simulink model "NucleoRespirator"  (R2018b)
settings: Solver=FixedStepDiscrete  StartTime=0.0  StopTime=10.0  FixedStep=MdlTS  RelTol=1e-3  SampleTimeConstraint=Specified  EnableMultiTasking=on
undefined symbols (not defined in the file): eSupervisorStates, NLCDDisplayColumns, ReleaseVersionMajor, ReleaseVersionMinor, ReleaseVersionRevision, tControlPeriod, tDisplayUpdatePeriode
libraries: RespiratorCtrlLib x37, simulink x4, LIB_Control x1
settings Model: DataDictionary=RespiratorControlData.sldd  ExtModeTrigDuration=10  Creator=BRAUL  LastModifiedBy=BRAUL
settings OptimizationCC: EnhancedBackFolding=on  PassReuseOutputArgsAs=Individual arguments  MaxStackSize=64  OptimizeBlockOrder=speed  DifferentSizesBufferReuse=on  OptimizationCustomize=off
settings DebuggingCC: UnderspecifiedInitializationDetection=Classic  MergeDetectMultiDrivingBlocksExec=none  ParameterTunabilityLossMsg=error
settings HardwareCC: ProdBitPerPointer=32  ProdBitPerSizeT=32  ProdBitPerPtrDiffT=32  ProdLargestAtomicInteger=Long  ProdLargestAtomicFloat=Double  ProdWordSize=32  ProdHWDeviceType=ARM Compatible->ARM Cortex
settings ModelReferenceCC: PropagateSignalLabelsOutOfModel=off
settings SFSimCC: MATLABDynamicMemAlloc=off
settings RTWCC: SystemTargetFile=ert.tlc  HardwareBoard=STM32 Nucleo F411RE  PackageGeneratedCodeAndArtifacts=on  TemplateMakefile=ert_default_tmf  GenerateReport=on  Toolchain=GNU Tools for ARM Embedded Processors  BuildConfiguration=Faster Runs  IncludeHyperlinkInReport=on  LaunchReport=on  GenerateTraceInfo=on  GenerateTraceReport=on  GenerateTraceReportSl=on  GenerateTraceReportSf=on  GenerateTraceReportEml=on  GenerateCodeReplacementReport=on
settings CodeAppCC: ForceParamTrailComments=on  IgnoreCustomStorageClasses=off  OperatorAnnotations=on  SimulinkDataObjDesc=on  SFDataObjDesc=on  InsertBlockDesc=on
settings ERTTargetCC: TargetLangStandard=C99 (ISO)  GenerateASAP2=on

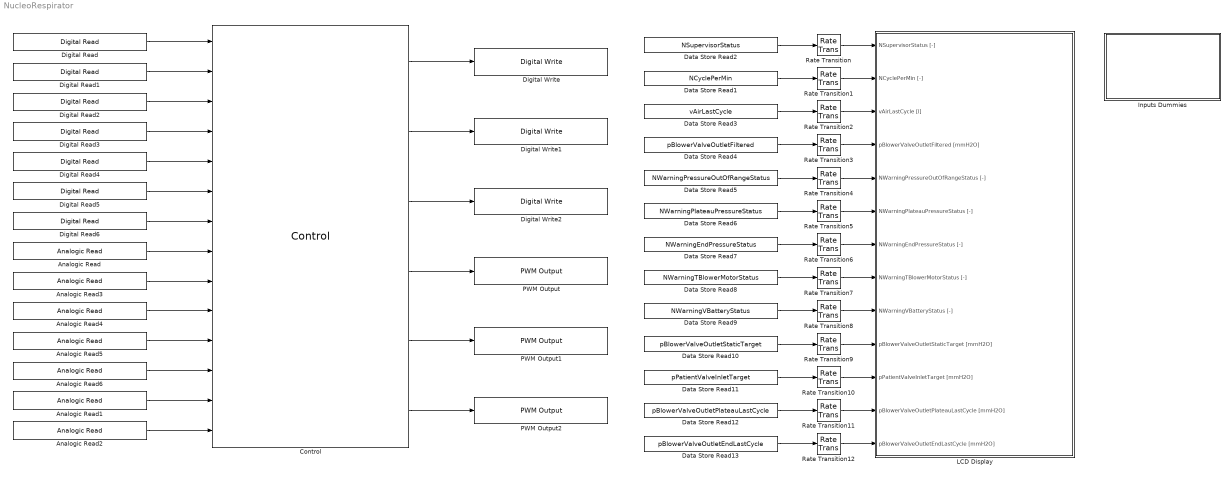
== system NucleoRespirator ==
  Analogic Read : RespiratorCtrlLib/Inputs/Analogic Read  pinFunc=pAir  pinSelected=PA_1  TS=-1
  Analogic Read1 : RespiratorCtrlLib/Inputs/Analogic Read  pinFunc=Motor Temp  pinSelected=PC_1  TS=-1
  Analogic Read2 : RespiratorCtrlLib/Inputs/Analogic Read  pinFunc=VBattery  pinSelected=PA_4  TS=-1
  Analogic Read3 : RespiratorCtrlLib/Inputs/Analogic Read  pinFunc=pStat QIn  pinSelected=PC_0  TS=-1
  Analogic Read4 : RespiratorCtrlLib/Inputs/Analogic Read  pinFunc=pDiff QIn  pinSelected=PA_0  TS=-1
  Analogic Read5 : RespiratorCtrlLib/Inputs/Analogic Read  pinFunc=pStat QOut  pinSelected=PB_0  TS=-1
  Analogic Read6 : RespiratorCtrlLib/Inputs/Analogic Read  pinFunc=pDiff QOut  pinSelected=PC_5  TS=-1
  Control : LIB_Control/Control  SystemSampleTime=tControlPeriod
      settings: AttributesFormatString=%<ReferenceBlock>
  Data Store Read1 : DataStoreRead  DataStoreName=NCyclePerMin  SampleTime=tControlPeriod
  Data Store Read10 : DataStoreRead  DataStoreName=pBlowerValveOutletStaticTarget  SampleTime=tControlPeriod
  Data Store Read11 : DataStoreRead  DataStoreName=pPatientValveInletTarget  SampleTime=tControlPeriod
  Data Store Read12 : DataStoreRead  DataStoreName=pBlowerValveOutletPlateauLastCycle  SampleTime=tControlPeriod
  Data Store Read13 : DataStoreRead  DataStoreName=pBlowerValveOutletEndLastCycle  SampleTime=tControlPeriod
  Data Store Read2 : DataStoreRead  DataStoreName=NSupervisorStatus  SampleTime=tControlPeriod
  Data Store Read3 : DataStoreRead  DataStoreName=vAirLastCycle  SampleTime=tControlPeriod
  Data Store Read4 : DataStoreRead  DataStoreName=pBlowerValveOutletFiltered  SampleTime=tControlPeriod
  Data Store Read5 : DataStoreRead  DataStoreName=NWarningPressureOutOfRangeStatus  SampleTime=tControlPeriod
  Data Store Read6 : DataStoreRead  DataStoreName=NWarningPlateauPressureStatus  SampleTime=tControlPeriod
  Data Store Read7 : DataStoreRead  DataStoreName=NWarningEndPressureStatus  SampleTime=tControlPeriod
  Data Store Read8 : DataStoreRead  DataStoreName=NWarningTBlowerMotorStatus  SampleTime=tControlPeriod
  Data Store Read9 : DataStoreRead  DataStoreName=NWarningVBatteryStatus  SampleTime=tControlPeriod
  Digital Read : RespiratorCtrlLib/Inputs/Digital Read  pinFunc=Start button  pinSelected=PC_13  TS=-1
  Digital Read1 : RespiratorCtrlLib/Inputs/Digital Read  pinFunc=Stop button  pinSelected=PB_15  TS=-1
  Digital Read2 : RespiratorCtrlLib/Inputs/Digital Read  pinFunc=Alam off button  pinSelected=PB_2  TS=-1
  Digital Read3 : RespiratorCtrlLib/Inputs/Digital Read  pinFunc=Service button  pinSelected=PB_12  TS=-1
  Digital Read4 : RespiratorCtrlLib/Inputs/Digital Read  pinFunc=Keyboard row 1  pinSelected=PC_9  TS=-1
  Digital Read5 : RespiratorCtrlLib/Inputs/Digital Read  pinFunc=Keyboard row 2  pinSelected=PC_10  TS=-1
  Digital Read6 : RespiratorCtrlLib/Inputs/Digital Read  pinFunc=Keyboard row 3  pinSelected=PC_11  TS=-1
  Digital Write : RespiratorCtrlLib/Outputs/Digital Write  pinFunc=Keyboard column 1  pinSelected=PC_2
  Digital Write1 : RespiratorCtrlLib/Outputs/Digital Write  pinFunc=Keyboard column 2  pinSelected=PC_3
  Digital Write2 : RespiratorCtrlLib/Outputs/Digital Write  pinFunc=Keyboard column 3  pinSelected=PC_6
  Inputs Dummies : Subsystem
  LCD Display : Subsystem  TreatAsAtomicUnit=on  SystemSampleTime=tDisplayUpdatePeriode
  PWM Output : RespiratorCtrlLib/Outputs/PWM Output  pinFunc=Blower Motor  pinSelected=PA_10  pwmFreq=fValvePwmFrequency
  PWM Output1 : RespiratorCtrlLib/Outputs/PWM Output  pinFunc=Blower Valve  pinSelected=PB_4  pwmFreq=fValvePwmFrequency
  PWM Output2 : RespiratorCtrlLib/Outputs/PWM Output  pinFunc=Patient Valve  pinSelected=PB_5  pwmFreq=fValvePwmFrequency
  Rate Transition{,1..12} (13 alike) : RateTransition
  wires:
  Analogic Read/1 -> Control/8
  Control/4 -> PWM Output/1
  Control/5 -> PWM Output1/1
  Control/6 -> PWM Output2/1
  Digital Read/1 -> Control/1
  Digital Read1/1 -> Control/2
  Digital Read2/1 -> Control/3
  Digital Read3/1 -> Control/4
  Analogic Read1/1 -> Control/13
  Analogic Read2/1 -> Control/14
  Digital Read4/1 -> Control/5
  Digital Read5/1 -> Control/6
  Digital Read6/1 -> Control/7
  Control/1 -> Digital Write/1
  Control/2 -> Digital Write1/1
  Control/3 -> Digital Write2/1
  Analogic Read3/1 -> Control/9
  Analogic Read4/1 -> Control/10
  Analogic Read5/1 -> Control/11
  Analogic Read6/1 -> Control/12
  Data Store Read2/1 -> Rate Transition/1
  Data Store Read1/1 -> Rate Transition1/1
  Data Store Read3/1 -> Rate Transition2/1
  Data Store Read4/1 -> Rate Transition3/1
  Data Store Read5/1 -> Rate Transition4/1
  Data Store Read6/1 -> Rate Transition5/1
  Data Store Read7/1 -> Rate Transition6/1
  Data Store Read8/1 -> Rate Transition7/1
  Data Store Read9/1 -> Rate Transition8/1
  Data Store Read10/1 -> Rate Transition9/1
  Data Store Read11/1 -> Rate Transition10/1
  Data Store Read12/1 -> Rate Transition11/1
  Data Store Read13/1 -> Rate Transition12/1
  Rate Transition/1 -> LCD Display/1(NSupervisorStatus [-])
  Rate Transition1/1 -> LCD Display/2(NCyclePerMin [-])
  Rate Transition2/1 -> LCD Display/3(vAirLastCycle [l])
  Rate Transition3/1 -> LCD Display/4(pBlowerValveOutletFiltered [mmH2O])
  Rate Transition4/1 -> LCD Display/5(NWarningPressureOutOfRangeStatus [-])
  Rate Transition5/1 -> LCD Display/6(NWarningPlateauPressureStatus [-])
  Rate Transition6/1 -> LCD Display/7(NWarningEndPressureStatus [-])
  Rate Transition7/1 -> LCD Display/8(NWarningTBlowerMotorStatus [-])
  Rate Transition8/1 -> LCD Display/9(NWarningVBatteryStatus [-])
  Rate Transition9/1 -> LCD Display/10(pBlowerValveOutletStaticTarget [mmH2O])
  Rate Transition10/1 -> LCD Display/11(pPatientValveInletTarget [mmH2O])
  Rate Transition11/1 -> LCD Display/12(pBlowerValveOutletPlateauLastCycle [mmH2O])
  Rate Transition12/1 -> LCD Display/13(pBlowerValveOutletEndLastCycle [mmH2O])

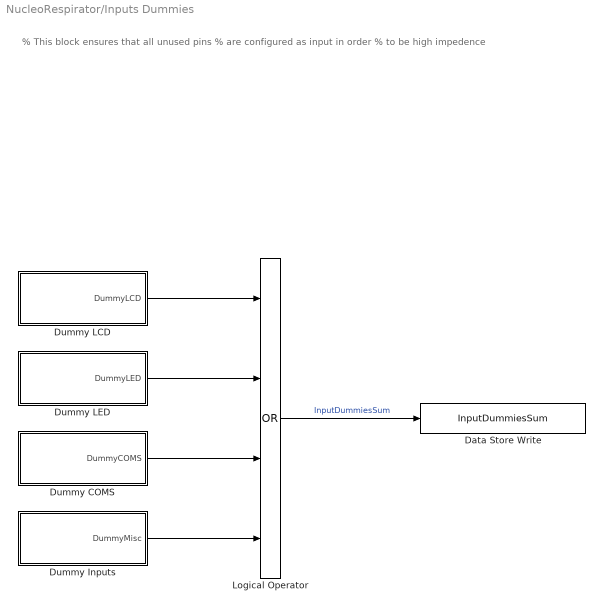
== system NucleoRespirator/Inputs Dummies ==
  note: % This block ensures that all unused pins
      | % are configured as input in order
      | % to be high impedence
  Data Store Write : DataStoreWrite  DataStoreName=InputDummiesSum
  Dummy COMS : Subsystem
  Dummy Inputs : Subsystem
  Dummy LCD : Subsystem
  Dummy LED : Subsystem
  Logical Operator : Logic  Operator=OR  Inputs=4  AllPortsSameDT=off  OutDataTypeStr=boolean
  wires:
  Dummy LCD/1(DummyLCD) -> Logical Operator/1
  Dummy LED/1(DummyLED) -> Logical Operator/2
  Dummy COMS/1(DummyCOMS) -> Logical Operator/3
  Dummy Inputs/1(DummyMisc) -> Logical Operator/4
  Logical Operator/1 -> Data Store Write/1  "InputDummiesSum"

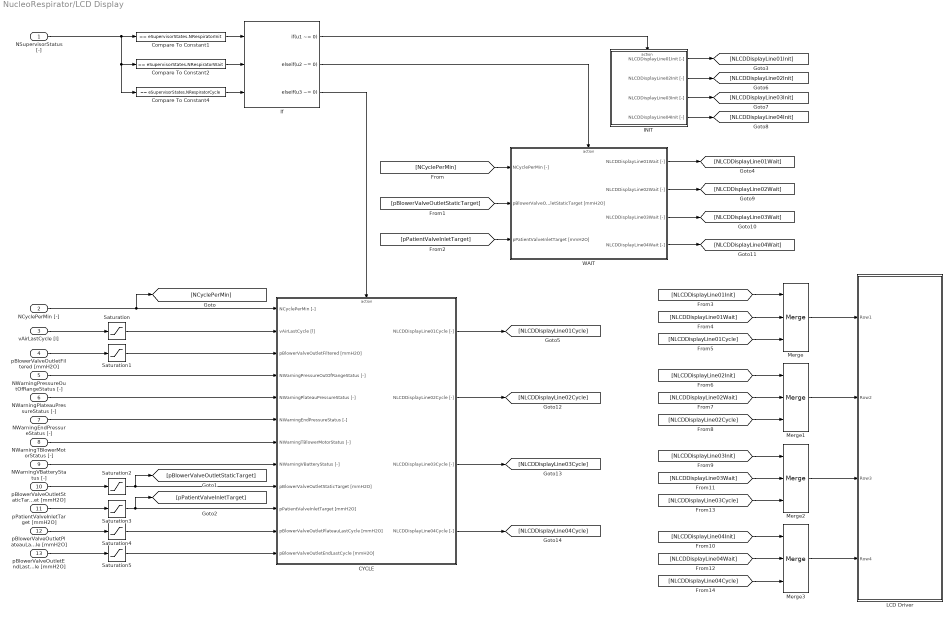
== system NucleoRespirator/LCD Display ==
  NSupervisorStatus [-] : Inport
  NCyclePerMin [-] : Inport  Port=2
  vAirLastCycle [l] : Inport  Port=3
  pBlowerValveOutletFiltered [mmH2O] : Inport  Port=4
  NWarningPressureOutOfRangeStatus [-] : Inport  Port=5
  NWarningPlateauPressureStatus [-] : Inport  Port=6
  NWarningEndPressureStatus [-] : Inport  Port=7
  NWarningTBlowerMotorStatus [-] : Inport  Port=8
  NWarningVBatteryStatus [-] : Inport  Port=9
  pBlowerValveOutletStaticTarget [mmH2O] : Inport  Port=10
  pPatientValveInletTarget [mmH2O] : Inport  Port=11
  pBlowerValveOutletPlateauLastCycle [mmH2O] : Inport  Port=12
  pBlowerValveOutletEndLastCycle [mmH2O] : Inport  Port=13
  CYCLE : Subsystem
  Compare To Constant1 : simulink/Logic and Bit Operations/Compare To Constant  relop===  const=eSupervisorStates.NRespiratorInit  OutDataTypeStr=boolean
  Compare To Constant2 : simulink/Logic and Bit Operations/Compare To Constant  relop===  const=eSupervisorStates.NRespiratorWait  OutDataTypeStr=boolean
  Compare To Constant4 : simulink/Logic and Bit Operations/Compare To Constant  relop===  const=eSupervisorStates.NRespiratorCycle  OutDataTypeStr=boolean
  INIT : Subsystem
  If : If  NumInputs=3  IfExpression=u1 ~= 0  ElseIfExpressions=u2 ~= 0,u3 ~= 0  ShowElse=off
  LCD Driver : Subsystem
  Merge{,1..3} (4 alike) : Merge  Inputs=3
  Saturation{,1..5} (6 alike) : Saturate  UpperLimit=inf  LowerLimit=0
  WAIT : Subsystem
  wires:
  Merge/1 -> LCD Driver/1(Row1)
  NWarningVBatteryStatus [-]/1 -> CYCLE/8(NWarningVBatteryStatus [-])
  NWarningTBlowerMotorStatus [-]/1 -> CYCLE/7(NWarningTBlowerMotorStatus [-])
  NWarningEndPressureStatus [-]/1 -> CYCLE/6(NWarningEndPressureStatus [-])
  NWarningPlateauPressureStatus [-]/1 -> CYCLE/5(NWarningPlateauPressureStatus [-])
  NWarningPressureOutOfRangeStatus [-]/1 -> CYCLE/4(NWarningPressureOutOfRangeStatus [-])
  [NLCDDisplayLine04Cycle] -> Merge3/3
  [NLCDDisplayLine03Cycle] -> Merge2/3
  [NLCDDisplayLine04Wait] -> Merge3/2
  [NLCDDisplayLine03Wait] -> Merge2/2
  [NLCDDisplayLine04Init] -> Merge3/1
  [NLCDDisplayLine03Init] -> Merge2/1
  [NLCDDisplayLine02Cycle] -> Merge1/3
  [NLCDDisplayLine02Wait] -> Merge1/2
  [NLCDDisplayLine02Init] -> Merge1/1
  [NLCDDisplayLine01Wait] -> Merge/2
  [NLCDDisplayLine01Init] -> Merge/1
  CYCLE/4(NLCDDisplayLine04Cycle [-]) -> [NLCDDisplayLine04Cycle]
  CYCLE/3(NLCDDisplayLine03Cycle [-]) -> [NLCDDisplayLine03Cycle]
  CYCLE/2(NLCDDisplayLine02Cycle [-]) -> [NLCDDisplayLine02Cycle]
  CYCLE/1(NLCDDisplayLine01Cycle [-]) -> [NLCDDisplayLine01Cycle]
  WAIT/4(NLCDDisplayLine04Wait [-]) -> [NLCDDisplayLine04Wait]
  WAIT/3(NLCDDisplayLine03Wait [-]) -> [NLCDDisplayLine03Wait]
  WAIT/2(NLCDDisplayLine02Wait [-]) -> [NLCDDisplayLine02Wait]
  INIT/4(NLCDDisplayLine04Init [-]) -> [NLCDDisplayLine04Init]
  INIT/3(NLCDDisplayLine03Init [-]) -> [NLCDDisplayLine03Init]
  WAIT/1(NLCDDisplayLine01Wait [-]) -> [NLCDDisplayLine01Wait]
  INIT/2(NLCDDisplayLine02Init [-]) -> [NLCDDisplayLine02Init]
  INIT/1(NLCDDisplayLine01Init [-]) -> [NLCDDisplayLine01Init]
  Merge3/1 -> LCD Driver/4(Row4)
  Merge2/1 -> LCD Driver/3(Row3)
  Merge1/1 -> LCD Driver/2(Row2)
  [pPatientValveInletTarget] -> WAIT/3(pPatientValveInletTarget [mmH2O])
  [pBlowerValveOutletStaticTarget] -> WAIT/2(pBlowerValveOutletStaticTarget [mmH2O])
  [NCyclePerMin] -> WAIT/1(NCyclePerMin [-])
  pBlowerValveOutletPlateauLastCycle [mmH2O]/1 -> Saturation4/1
  pBlowerValveOutletEndLastCycle [mmH2O]/1 -> Saturation5/1
  pBlowerValveOutletFiltered [mmH2O]/1 -> Saturation1/1
  vAirLastCycle [l]/1 -> Saturation/1
  pPatientValveInletTarget [mmH2O]/1 -> Saturation3/1
  pBlowerValveOutletStaticTarget [mmH2O]/1 -> Saturation2/1
  NCyclePerMin [-]/1 -> CYCLE/1(NCyclePerMin [-]), [NCyclePerMin]
  If/2 -> WAIT/Action
  Compare To Constant2/1 -> If/2
  Compare To Constant4/1 -> If/3
  NSupervisorStatus [-]/1 -> Compare To Constant1/1, Compare To Constant4/1, Compare To Constant2/1
  If/3 -> CYCLE/Action
  Compare To Constant1/1 -> If/1
  If/1 -> INIT/Action
  [NLCDDisplayLine01Cycle] -> Merge/3
  Saturation/1 -> CYCLE/2(vAirLastCycle [l])
  Saturation1/1 -> CYCLE/3(pBlowerValveOutletFiltered [mmH2O])
  Saturation2/1 -> CYCLE/9(pBlowerValveOutletStaticTarget [mmH2O]), [pBlowerValveOutletStaticTarget]
  Saturation3/1 -> CYCLE/10(pPatientValveInletTarget [mmH2O]), [pPatientValveInletTarget]
  Saturation4/1 -> CYCLE/11(pBlowerValveOutletPlateauLastCycle [mmH2O])
  Saturation5/1 -> CYCLE/12(pBlowerValveOutletEndLastCycle [mmH2O])

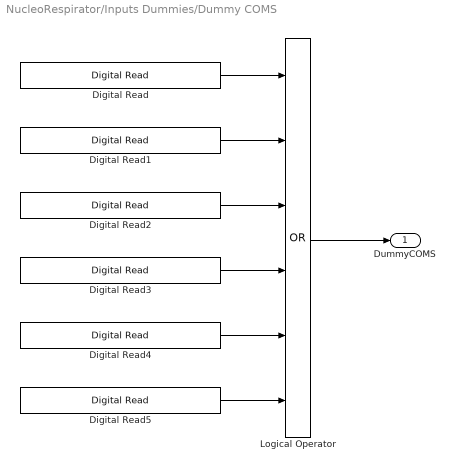
== system NucleoRespirator/Inputs Dummies/Dummy COMS ==
  Digital Read : RespiratorCtrlLib/Inputs/Digital Read  pinFunc=Dummy UART1 TX  pinSelected=PA_9  TS=-1
  Digital Read1 : RespiratorCtrlLib/Inputs/Digital Read  pinFunc=Dummy UART1 RX  pinSelected=PB_3  TS=-1
  Digital Read2 : RespiratorCtrlLib/Inputs/Digital Read  pinFunc=Dummy SCI6 TX  pinSelected=PA_11  TS=-1
  Digital Read3 : RespiratorCtrlLib/Inputs/Digital Read  pinFunc=Dummy SCI6 RX  pinSelected=PA_12  TS=-1
  Digital Read4 : RespiratorCtrlLib/Inputs/Digital Read  pinFunc=Dummy I2C1 SCL  pinSelected=PB_8  TS=-1
  Digital Read5 : RespiratorCtrlLib/Inputs/Digital Read  pinFunc=Dummy I2C1 SDA  pinSelected=PB_9  TS=-1
  Logical Operator : Logic  Operator=OR  Inputs=6  AllPortsSameDT=off  OutDataTypeStr=boolean
  DummyCOMS : Outport
  wires:
  Logical Operator/1 -> DummyCOMS/1
  Digital Read/1 -> Logical Operator/1
  Digital Read1/1 -> Logical Operator/2
  Digital Read2/1 -> Logical Operator/3
  Digital Read3/1 -> Logical Operator/4
  Digital Read5/1 -> Logical Operator/6
  Digital Read4/1 -> Logical Operator/5

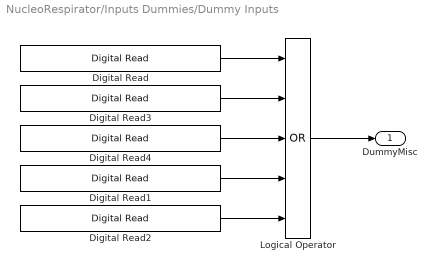
== system NucleoRespirator/Inputs Dummies/Dummy Inputs ==
  Digital Read : RespiratorCtrlLib/Inputs/Digital Read  pinFunc=Dummy In Tachy  pinSelected=PA_15  TS=-1
  Digital Read1 : RespiratorCtrlLib/Inputs/Digital Read  pinFunc=Dummy Expander1  pinSelected=PB_1  TS=-1
  Digital Read2 : RespiratorCtrlLib/Inputs/Digital Read  pinFunc=Dummy Expander2  pinSelected=PB_6  TS=-1
  Digital Read3 : RespiratorCtrlLib/Inputs/Digital Read  pinFunc=Dummy FLT_ADM  pinSelected=PC_14  TS=-1
  Digital Read4 : RespiratorCtrlLib/Inputs/Digital Read  pinFunc=Dummy FLT_ECH  pinSelected=PC_15  TS=-1
  Logical Operator : Logic  Operator=OR  Inputs=5  AllPortsSameDT=off  OutDataTypeStr=boolean
  DummyMisc : Outport
  wires:
  Digital Read/1 -> Logical Operator/1
  Digital Read3/1 -> Logical Operator/2
  Digital Read4/1 -> Logical Operator/3
  Digital Read1/1 -> Logical Operator/4
  Digital Read2/1 -> Logical Operator/5
  Logical Operator/1 -> DummyMisc/1

== system NucleoRespirator/Inputs Dummies/Dummy LCD ==
  Digital Read7 : RespiratorCtrlLib/Inputs/Digital Read  pinFunc=Dummy Buzzer  pinSelected=PB_7  TS=-1
  DummyLCD : Outport
  wires:
  Digital Read7/1 -> DummyLCD/1

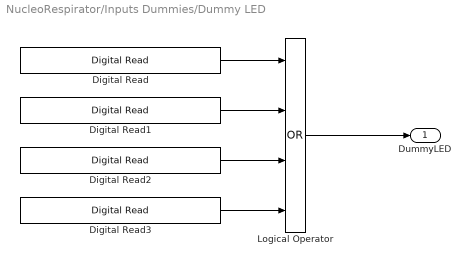
== system NucleoRespirator/Inputs Dummies/Dummy LED ==
  Digital Read : RespiratorCtrlLib/Inputs/Digital Read  pinFunc=Dummy LED Start  pinSelected=PC_8  TS=-1
  Digital Read1 : RespiratorCtrlLib/Inputs/Digital Read  pinFunc=Dummy LED Alaram  pinSelected=PB_13  TS=-1
  Digital Read2 : RespiratorCtrlLib/Inputs/Digital Read  pinFunc=Dummy LED Alaram MED  pinSelected=PB_14  TS=-1
  Digital Read3 : RespiratorCtrlLib/Inputs/Digital Read  pinFunc=Dummy LED Alaram High  pinSelected=PC_4  TS=-1
  Logical Operator : Logic  Operator=OR  Inputs=4  AllPortsSameDT=off  OutDataTypeStr=boolean
  DummyLED : Outport
  wires:
  Logical Operator/1 -> DummyLED/1
  Digital Read2/1 -> Logical Operator/3
  Digital Read1/1 -> Logical Operator/2
  Digital Read/1 -> Logical Operator/1
  Digital Read3/1 -> Logical Operator/4

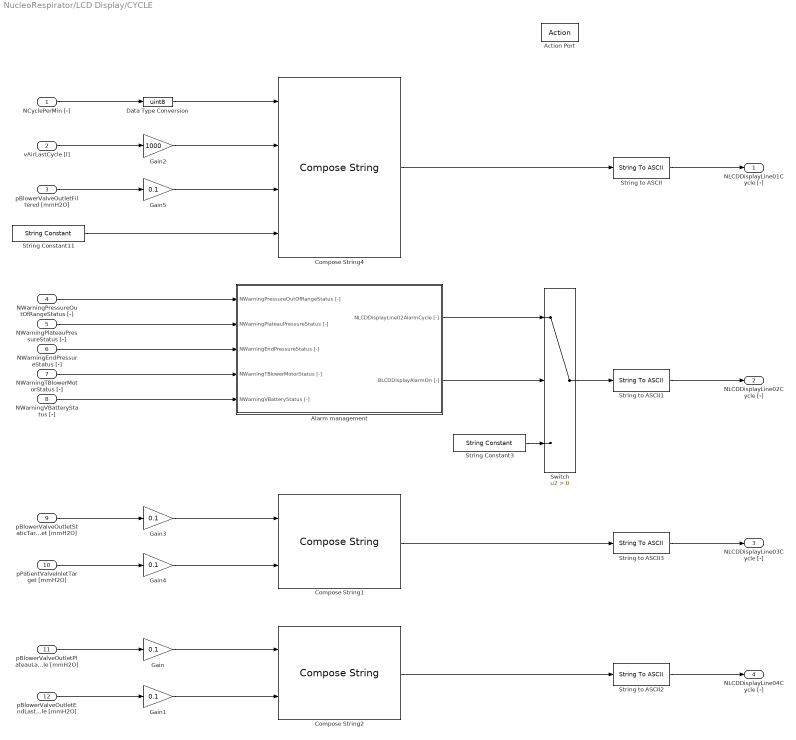
== system NucleoRespirator/LCD Display/CYCLE ==
  NCyclePerMin [-] : Inport
  vAirLastCycle [l] : Inport  Port=2
  pBlowerValveOutletFiltered [mmH2O] : Inport  Port=3
  NWarningPressureOutOfRangeStatus [-] : Inport  Port=4
  NWarningPlateauPressureStatus [-] : Inport  Port=5
  NWarningEndPressureStatus [-] : Inport  Port=6
  NWarningTBlowerMotorStatus [-] : Inport  Port=7
  NWarningVBatteryStatus [-] : Inport  Port=8
  pBlowerValveOutletStaticTarget [mmH2O] : Inport  Port=9
  pPatientValveInletTarget [mmH2O] : Inport  Port=10
  pBlowerValveOutletPlateauLastCycle [mmH2O] : Inport  Port=11
  pBlowerValveOutletEndLastCycle [mmH2O] : Inport  Port=12
  Action Port : ActionPort  ActionType=elseif
  Alarm management : Subsystem
  Compose String1 : ComposeString  Format="\"set:  %02u     %02u   cm\""
  Compose String2 : ComposeString  Format="\"meas: %02u     %02u   cm\""
  Compose String4 : ComposeString  Format="\"%02ucpm %03uml %02ucm %2s%%%%\""
  Data Type Conversion : DataTypeConversion  OutDataTypeStr=uint8
  Gain{,1,3..5} (5 alike) : Gain  Description=mmH2O --> cmH2O  Gain=0.1  OutDataTypeStr=uint8
      settings: AttributesFormatString=|
      | %<Description>
      | %<OutDataTypeStr>
  Gain2 : Gain  Description=l --> ml  Gain=1000  OutDataTypeStr=uint16
      settings: AttributesFormatString=|
      | %<Description>
      | %<OutDataTypeStr>
  String Constant11 : StringConstant  Description=Taux O2  String='??'
      settings: AttributesFormatString=%<Description>
  String Constant3 : StringConstant  String="'      pINSP  pEEP'"
  String to ASCII{,1..3} (4 alike) : StringToASCII  MaximumLength=NLCDDisplayColumns+1
  Switch : Switch  Criteria=u2 > Threshold
  NLCDDisplayLine01Cycle [-] : Outport
  NLCDDisplayLine02Cycle [-] : Outport  Port=2
  NLCDDisplayLine03Cycle [-] : Outport  Port=3
  NLCDDisplayLine04Cycle [-] : Outport  Port=4
  wires:
  Switch/1 -> String to ASCII1/1
  String Constant3/1 -> Switch/3
  Alarm management/1(NLCDDisplayLine02AlarmCycle [-]) -> Switch/1
  Alarm management/2(BLCDDisplayAlarmOn [-]) -> Switch/2
  NWarningVBatteryStatus [-]/1 -> Alarm management/5(NWarningVBatteryStatus [-])
  NWarningTBlowerMotorStatus [-]/1 -> Alarm management/4(NWarningTBlowerMotorStatus [-])
  NWarningPressureOutOfRangeStatus [-]/1 -> Alarm management/1(NWarningPressureOutOfRangeStatus [-])
  NWarningEndPressureStatus [-]/1 -> Alarm management/3(NWarningEndPressureStatus [-])
  NWarningPlateauPressureStatus [-]/1 -> Alarm management/2(NWarningPlateauPressureStatus [-])
  pBlowerValveOutletEndLastCycle [mmH2O]/1 -> Gain1/1
  pBlowerValveOutletPlateauLastCycle [mmH2O]/1 -> Gain/1
  String Constant11/1 -> Compose String4/4
  pBlowerValveOutletFiltered [mmH2O]/1 -> Gain5/1
  Compose String1/1 -> String to ASCII3/1
  Gain3/1 -> Compose String1/1
  Gain4/1 -> Compose String1/2
  Gain5/1 -> Compose String4/3
  Gain2/1 -> Compose String4/2
  vAirLastCycle [l]/1 -> Gain2/1
  String to ASCII1/1 -> NLCDDisplayLine02Cycle [-]/1
  String to ASCII/1 -> NLCDDisplayLine01Cycle [-]/1
  NCyclePerMin [-]/1 -> Data Type Conversion/1
  String to ASCII2/1 -> NLCDDisplayLine04Cycle [-]/1
  Compose String2/1 -> String to ASCII2/1
  pBlowerValveOutletStaticTarget [mmH2O]/1 -> Gain3/1
  pPatientValveInletTarget [mmH2O]/1 -> Gain4/1
  String to ASCII3/1 -> NLCDDisplayLine03Cycle [-]/1
  Gain/1 -> Compose String2/1
  Gain1/1 -> Compose String2/2
  Data Type Conversion/1 -> Compose String4/1
  Compose String4/1 -> String to ASCII/1

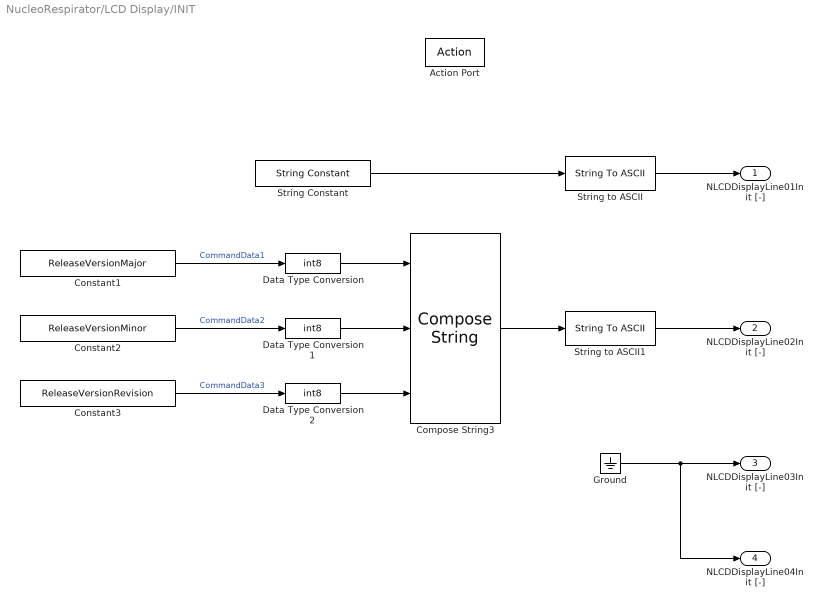
== system NucleoRespirator/LCD Display/INIT ==
  Action Port : ActionPort  ActionType=then
  Compose String3 : ComposeString  Format="\"v%d.%d.%d\""
  Constant1 : Constant  Value=ReleaseVersionMajor  OutDataTypeStr=uint8
  Constant2 : Constant  Value=ReleaseVersionMinor  OutDataTypeStr=uint8
  Constant3 : Constant  Value=ReleaseVersionRevision  OutDataTypeStr=uint8
  Data Type Conversion : DataTypeConversion  OutDataTypeStr=int8
  Data Type Conversion1 : DataTypeConversion  OutDataTypeStr=int8
  Data Type Conversion2 : DataTypeConversion  OutDataTypeStr=int8
  Ground : Ground
  String Constant : StringConstant  String='Initialization'
  String to ASCII : StringToASCII  MaximumLength=NLCDDisplayColumns+1
  String to ASCII1 : StringToASCII  MaximumLength=NLCDDisplayColumns+1
  NLCDDisplayLine01Init [-] : Outport
  NLCDDisplayLine02Init [-] : Outport  Port=2
  NLCDDisplayLine03Init [-] : Outport  Port=3
  NLCDDisplayLine04Init [-] : Outport  Port=4
  wires:
  String to ASCII1/1 -> NLCDDisplayLine02Init [-]/1
  String to ASCII/1 -> NLCDDisplayLine01Init [-]/1
  Compose String3/1 -> String to ASCII1/1
  Constant3/1 -> Data Type Conversion2/1  "CommandData3"
  Constant2/1 -> Data Type Conversion1/1  "CommandData2"
  Constant1/1 -> Data Type Conversion/1  "CommandData1"
  Data Type Conversion/1 -> Compose String3/1
  String Constant/1 -> String to ASCII/1
  Data Type Conversion1/1 -> Compose String3/2
  Data Type Conversion2/1 -> Compose String3/3
  Ground/1 -> NLCDDisplayLine04Init [-]/1, NLCDDisplayLine03Init [-]/1

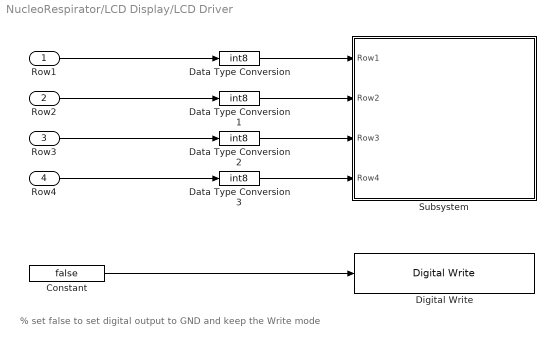
== system NucleoRespirator/LCD Display/LCD Driver ==
  note: % set false to set digital output to GND and keep the Write mode
  Row1 : Inport
  Row2 : Inport  Port=2
  Row3 : Inport  Port=3
  Row4 : Inport  Port=4
  Constant : Constant  Value=false  OutDataTypeStr=boolean
  Data Type Conversion{,1..3} (4 alike) : DataTypeConversion  OutDataTypeStr=int8
  Digital Write : RespiratorCtrlLib/Outputs/Digital Write  pinFunc=LCD RW  pinSelected=PC_12
  Subsystem : Subsystem  mask{pRS=PA_8, pE=PA_5, pDB1=PC_7, pDB2=PB_10, pDB3=PA_7, pDB4=PA_6}
      mask prompts: pRS "RS Pin"; pE "Enable Pin"; pDB1 "Data bit 1 Pin"; pDB2 "Data bit 2 Pin"; pDB3 "Data bit 3 Pin"; pDB4 "Data bit 4 Pin"
      mask init:
      | initLcdDriver(gcb);
      settings: OpenFcn=|
      | setLcdPinNames(gcb);
      | open_system(gcb, 'mask');
      mask TypeOptions pRS: A0 | A1 | A2 | A3 | A4 | A5 | D0 | D1 | D2 | D3 | D4 | D5 | D6 | D7 | D8 | D9 | D10 | D11 | D12 | D13 | D14 | D15 | PA_0 | PA_1 | PA_2 | PA_3 | PA_4 | PA_5 | PA_6 | PA_7 | PA_8 | PA_9 | PA_10 | PA_11 | PA_12 | PA_13 | PA_14 | PA_15 | PB_0 | PB_1 | PB_2 | PB_3 | PB_4 | PB_5 | PB_6 | PB_7 | PB_8 | PB_9 | PB_10 | PB_11 | PB_12 | PB_13 | PB_14 | PB_15 | PC_0 | PC_1 | PC_2 | PC_3 | PC_4 | PC_5 | PC_6 | PC_7 | PC_8 | PC_9 | PC_10 | PC_11 | PC_12 | PC_13 | PC_14 | PC_15 | PD_2 | PH_0 | PH_1 | NC
      mask TypeOptions pE: A0 | A1 | A2 | A3 | A4 | A5 | D0 | D1 | D2 | D3 | D4 | D5 | D6 | D7 | D8 | D9 | D10 | D11 | D12 | D13 | D14 | D15 | PA_0 | PA_1 | PA_2 | PA_3 | PA_4 | PA_5 | PA_6 | PA_7 | PA_8 | PA_9 | PA_10 | PA_11 | PA_12 | PA_13 | PA_14 | PA_15 | PB_0 | PB_1 | PB_2 | PB_3 | PB_4 | PB_5 | PB_6 | PB_7 | PB_8 | PB_9 | PB_10 | PB_11 | PB_12 | PB_13 | PB_14 | PB_15 | PC_0 | PC_1 | PC_2 | PC_3 | PC_4 | PC_5 | PC_6 | PC_7 | PC_8 | PC_9 | PC_10 | PC_11 | PC_12 | PC_13 | PC_14 | PC_15 | PD_2 | PH_0 | PH_1 | NC
      mask TypeOptions pDB1: A0 | A1 | A2 | A3 | A4 | A5 | D0 | D1 | D2 | D3 | D4 | D5 | D6 | D7 | D8 | D9 | D10 | D11 | D12 | D13 | D14 | D15 | PA_0 | PA_1 | PA_2 | PA_3 | PA_4 | PA_5 | PA_6 | PA_7 | PA_8 | PA_9 | PA_10 | PA_11 | PA_12 | PA_13 | PA_14 | PA_15 | PB_0 | PB_1 | PB_2 | PB_3 | PB_4 | PB_5 | PB_6 | PB_7 | PB_8 | PB_9 | PB_10 | PB_11 | PB_12 | PB_13 | PB_14 | PB_15 | PC_0 | PC_1 | PC_2 | PC_3 | PC_4 | PC_5 | PC_6 | PC_7 | PC_8 | PC_9 | PC_10 | PC_11 | PC_12 | PC_13 | PC_14 | PC_15 | PD_2 | PH_0 | PH_1 | NC
      mask TypeOptions pDB2: A0 | A1 | A2 | A3 | A4 | A5 | D0 | D1 | D2 | D3 | D4 | D5 | D6 | D7 | D8 | D9 | D10 | D11 | D12 | D13 | D14 | D15 | PA_0 | PA_1 | PA_2 | PA_3 | PA_4 | PA_5 | PA_6 | PA_7 | PA_8 | PA_9 | PA_10 | PA_11 | PA_12 | PA_13 | PA_14 | PA_15 | PB_0 | PB_1 | PB_2 | PB_3 | PB_4 | PB_5 | PB_6 | PB_7 | PB_8 | PB_9 | PB_10 | PB_11 | PB_12 | PB_13 | PB_14 | PB_15 | PC_0 | PC_1 | PC_2 | PC_3 | PC_4 | PC_5 | PC_6 | PC_7 | PC_8 | PC_9 | PC_10 | PC_11 | PC_12 | PC_13 | PC_14 | PC_15 | PD_2 | PH_0 | PH_1 | NC
      mask TypeOptions pDB3: A0 | A1 | A2 | A3 | A4 | A5 | D0 | D1 | D2 | D3 | D4 | D5 | D6 | D7 | D8 | D9 | D10 | D11 | D12 | D13 | D14 | D15 | PA_0 | PA_1 | PA_2 | PA_3 | PA_4 | PA_5 | PA_6 | PA_7 | PA_8 | PA_9 | PA_10 | PA_11 | PA_12 | PA_13 | PA_14 | PA_15 | PB_0 | PB_1 | PB_2 | PB_3 | PB_4 | PB_5 | PB_6 | PB_7 | PB_8 | PB_9 | PB_10 | PB_11 | PB_12 | PB_13 | PB_14 | PB_15 | PC_0 | PC_1 | PC_2 | PC_3 | PC_4 | PC_5 | PC_6 | PC_7 | PC_8 | PC_9 | PC_10 | PC_11 | PC_12 | PC_13 | PC_14 | PC_15 | PD_2 | PH_0 | PH_1 | NC
      mask TypeOptions pDB4: A0 | A1 | A2 | A3 | A4 | A5 | D0 | D1 | D2 | D3 | D4 | D5 | D6 | D7 | D8 | D9 | D10 | D11 | D12 | D13 | D14 | D15 | PA_0 | PA_1 | PA_2 | PA_3 | PA_4 | PA_5 | PA_6 | PA_7 | PA_8 | PA_9 | PA_10 | PA_11 | PA_12 | PA_13 | PA_14 | PA_15 | PB_0 | PB_1 | PB_2 | PB_3 | PB_4 | PB_5 | PB_6 | PB_7 | PB_8 | PB_9 | PB_10 | PB_11 | PB_12 | PB_13 | PB_14 | PB_15 | PC_0 | PC_1 | PC_2 | PC_3 | PC_4 | PC_5 | PC_6 | PC_7 | PC_8 | PC_9 | PC_10 | PC_11 | PC_12 | PC_13 | PC_14 | PC_15 | PD_2 | PH_0 | PH_1 | NC
      mask Display: disp('LCD Display\nDriver\n\n   RS: PA_8\n     E: PA_5\n   D1: PC_7\n   D2: PB_10\n   D3: PA_7\n   D4: PA_6')
  wires:
  Data Type Conversion2/1 -> Subsystem/3(Row3)
  Row2/1 -> Data Type Conversion1/1
  Data Type Conversion3/1 -> Subsystem/4(Row4)
  Row3/1 -> Data Type Conversion2/1
  Constant/1 -> Digital Write/1
  Data Type Conversion/1 -> Subsystem/1(Row1)
  Data Type Conversion1/1 -> Subsystem/2(Row2)
  Row4/1 -> Data Type Conversion3/1
  Row1/1 -> Data Type Conversion/1

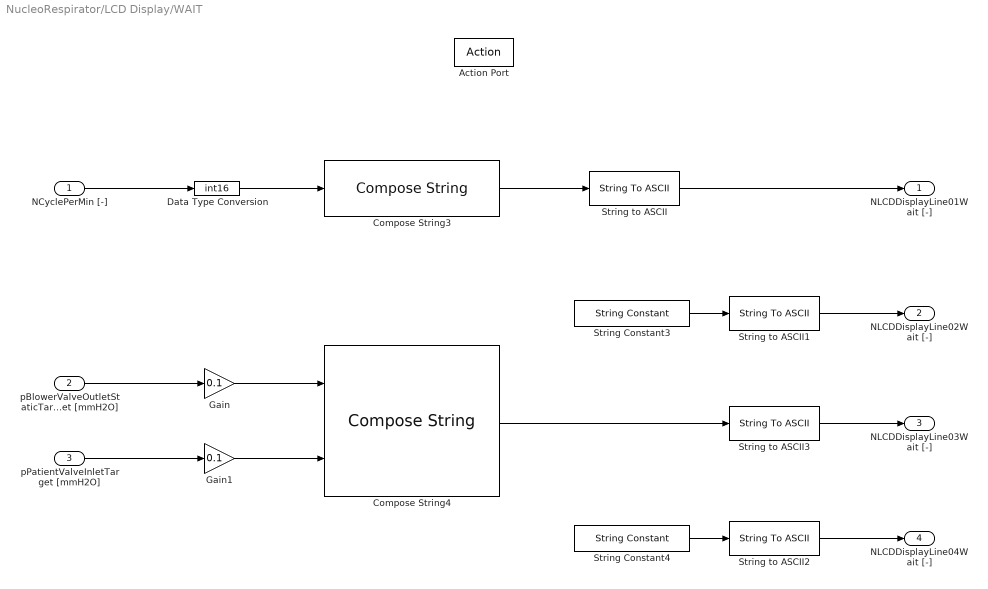
== system NucleoRespirator/LCD Display/WAIT ==
  NCyclePerMin [-] : Inport
  pBlowerValveOutletStaticTarget [mmH2O] : Inport  Port=2
  pPatientValveInletTarget [mmH2O] : Inport  Port=3
  Action Port : ActionPort  ActionType=elseif
  Compose String3 : ComposeString  Format="\"%02dcpm   0ml  0cm   %%%%\""
  Compose String4 : ComposeString  Format="\"set:  %02d     %02d   cm\""
  Data Type Conversion : DataTypeConversion  OutDataTypeStr=int16
  Gain : Gain  Description=mmH2O --> cmH2O  Gain=0.1  OutDataTypeStr=int16
      settings: AttributesFormatString=|
      | %<Description>
      | %<OutDataTypeStr>
  Gain1 : Gain  Description=mmH2O --> cmH2O  Gain=0.1  OutDataTypeStr=int16
      settings: AttributesFormatString=|
      | %<Description>
      | %<OutDataTypeStr>
  String Constant3 : StringConstant  String="'      pINSP  pEEP   '"
  String Constant4 : StringConstant  String='Press start to begin'
  String to ASCII{,1..3} (4 alike) : StringToASCII  MaximumLength=NLCDDisplayColumns+1
  NLCDDisplayLine01Wait [-] : Outport
  NLCDDisplayLine02Wait [-] : Outport  Port=2
  NLCDDisplayLine03Wait [-] : Outport  Port=3
  NLCDDisplayLine04Wait [-] : Outport  Port=4
  wires:
  Gain1/1 -> Compose String4/2
  Gain/1 -> Compose String4/1
  Compose String4/1 -> String to ASCII3/1
  String to ASCII3/1 -> NLCDDisplayLine03Wait [-]/1
  pPatientValveInletTarget [mmH2O]/1 -> Gain1/1
  pBlowerValveOutletStaticTarget [mmH2O]/1 -> Gain/1
  String Constant4/1 -> String to ASCII2/1
  String to ASCII2/1 -> NLCDDisplayLine04Wait [-]/1
  String Constant3/1 -> String to ASCII1/1
  String to ASCII/1 -> NLCDDisplayLine01Wait [-]/1
  String to ASCII1/1 -> NLCDDisplayLine02Wait [-]/1
  NCyclePerMin [-]/1 -> Data Type Conversion/1
  Data Type Conversion/1 -> Compose String3/1
  Compose String3/1 -> String to ASCII/1

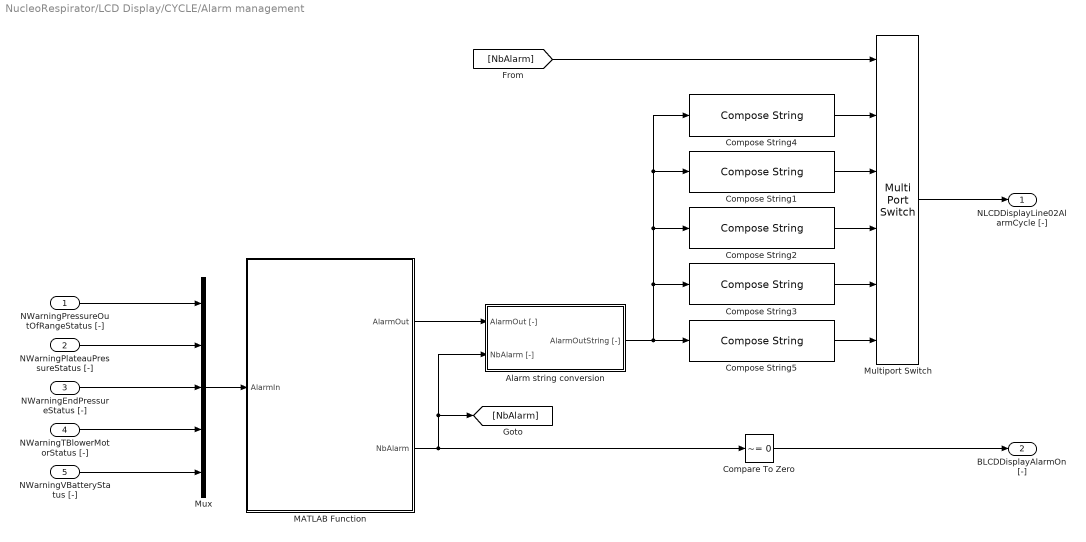
== system NucleoRespirator/LCD Display/CYCLE/Alarm management ==
  NWarningPressureOutOfRangeStatus [-] : Inport
  NWarningPlateauPressureStatus [-] : Inport  Port=2
  NWarningEndPressureStatus [-] : Inport  Port=3
  NWarningTBlowerMotorStatus [-] : Inport  Port=4
  NWarningVBatteryStatus [-] : Inport  Port=5
  Alarm string conversion : Subsystem
  Compare To Zero : simulink/Logic and Bit Operations/Compare To Zero  relop=~=  OutDataTypeStr=boolean
  Compose String1 : ComposeString  Format="\"Alarm: %5s        \""
  Compose String2 : ComposeString  Format="\"Alarm: %8s     \""
  Compose String3 : ComposeString  Format="\"Alarm: %11s  \""
  Compose String4 : ComposeString  Format="\"Alarm: %2s           \""
  Compose String5 : ComposeString  Format="\"Alarm:%14s\""
  MATLAB Function : MATLAB Function  TreatAsAtomicUnit=on
  Multiport Switch : MultiPortSwitch  Inputs=5
  Mux : Mux  Inputs=5
  NLCDDisplayLine02AlarmCycle [-] : Outport
  BLCDDisplayAlarmOn [-] : Outport  Port=2
  wires:
  MATLAB Function/2(NbAlarm) -> Alarm string conversion/2(NbAlarm [-]), [NbAlarm], Compare To Zero/1
  Alarm string conversion/1(AlarmOutString [-]) -> Compose String5/1, Compose String3/1, Compose String1/1, Compose String4/1, Compose String2/1
  MATLAB Function/1(AlarmOut) -> Alarm string conversion/1(AlarmOut [-])
  Multiport Switch/1 -> NLCDDisplayLine02AlarmCycle [-]/1
  [NbAlarm] -> Multiport Switch/1
  Compare To Zero/1 -> BLCDDisplayAlarmOn [-]/1
  NWarningVBatteryStatus [-]/1 -> Mux/5
  NWarningTBlowerMotorStatus [-]/1 -> Mux/4
  NWarningEndPressureStatus [-]/1 -> Mux/3
  NWarningPlateauPressureStatus [-]/1 -> Mux/2
  NWarningPressureOutOfRangeStatus [-]/1 -> Mux/1
  Mux/1 -> MATLAB Function/1(AlarmIn)
  Compose String4/1 -> Multiport Switch/2
  Compose String1/1 -> Multiport Switch/3
  Compose String2/1 -> Multiport Switch/4
  Compose String3/1 -> Multiport Switch/5
  Compose String5/1 -> Multiport Switch/6

== system NucleoRespirator/LCD Display/LCD Driver/Subsystem ==
  Row1 : Inport
  Row2 : Inport  Port=2
  Row3 : Inport  Port=3
  Row4 : Inport  Port=4
  TextLCD_System : MATLABSystem  System=DriverLCD  RS_Pin=int32(7)  Enable_Pin=int32(13)  Data_Pin1=int32(9)  Data_Pin2=int32(6)  Data_Pin3=int32(11)  Data_Pin4=int32(12)
      mask Type: DriverLCD
      mask Display:
      | disp('MBED\nTextLCD');
      | port_label('input',1,'Row1');
      | port_label('input',2,'Row2');
      | port_label('input',3,'Row3');
      | port_label('input',4,'Row4');
  wires:
  Row3/1 -> TextLCD_System/3
  Row2/1 -> TextLCD_System/2
  Row4/1 -> TextLCD_System/4
  Row1/1 -> TextLCD_System/1

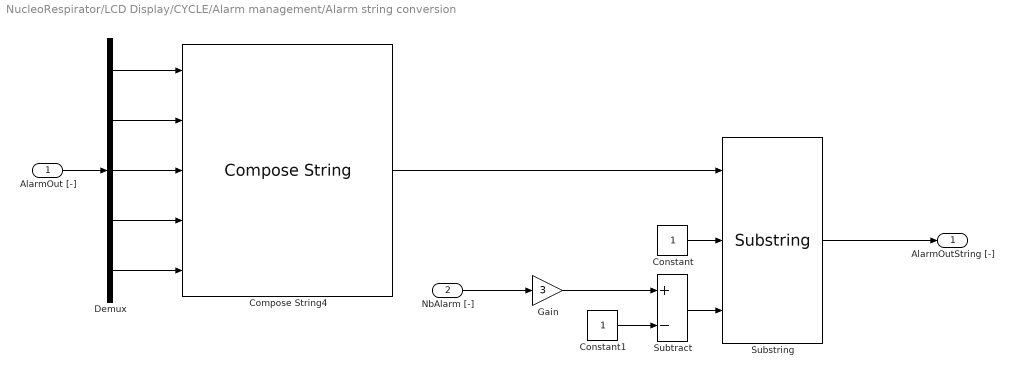
== system NucleoRespirator/LCD Display/CYCLE/Alarm management/Alarm string conversion ==
  AlarmOut [-] : Inport
  NbAlarm [-] : Inport  Port=2
  Compose String4 : ComposeString  Format="\"%02u %02u %02u %02u %02u\""
  Constant : Constant  OutDataTypeStr=uint8
  Constant1 : Constant  OutDataTypeStr=uint8
  Demux : Demux  Outputs=5
  Gain : Gain  Gain=3  OutDataTypeStr=uint8
  Substring : Substring
  Subtract : Sum  Inputs=+-
  AlarmOutString [-] : Outport
  wires:
  Constant1/1 -> Subtract/2
  NbAlarm [-]/1 -> Gain/1
  Gain/1 -> Subtract/1
  Subtract/1 -> Substring/3
  Substring/1 -> AlarmOutString [-]/1
  Constant/1 -> Substring/2
  Compose String4/1 -> Substring/1
  Demux/4 -> Compose String4/4
  Demux/5 -> Compose String4/5
  Demux/3 -> Compose String4/3
  Demux/1 -> Compose String4/1
  AlarmOut [-]/1 -> Demux/1
  Demux/2 -> Compose String4/2

== matlab function NucleoRespirator/LCD Display/CYCLE/Alarm management/MATLAB Function ==
  data: AlarmIn input uint8; AlarmOut output uint8; NbAlarm output uint8
function [AlarmOut,NbAlarm] = AlarmSorting(AlarmIn)

NbAlarm = uint8(0);
AlarmOn = uint8(99*ones(1,5));

for i=1:5
    if AlarmIn(i) ~= 0
        NbAlarm = NbAlarm + 1;
        AlarmOn(NbAlarm) = AlarmIn(i);
    end
end
AlarmOut = uint8(99*ones(1,5));
for i=1:NbAlarm
    [AlarmMin,IndexMin] = min(AlarmOn);
    AlarmOut(i) = AlarmMin;
    AlarmOn(IndexMin) = 99;
end
